simulink model "Sys1"  (R2017b)
settings: Solver=VariableStepAuto  StartTime=0.0  StopTime=10.0  RelTol=1e-3
values from neighbouring files (symbols this model uses):
  Gs_Ident = tf([-0.01542 5.826],[1 1.226])    [main.m]
libraries: simulink x1
settings Model: Creator=felip  LastModifiedBy=felip

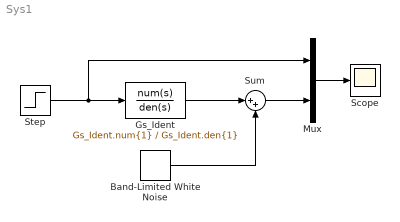
== system Sys1 ==
  Band-Limited White Noise : simulink/Sources/Band-Limited White Noise  Cov=1e-7  Ts=1e-3  seed=[23341]
  Gs_Ident : TransferFcn  Numerator=Gs_Ident.num{1}  Denominator=Gs_Ident.den{1}
  Mux : Mux  Inputs=2
  Scope : Scope
  Step : Step  SampleTime=0
  Sum : Sum  Inputs=|++
  wires:
  Step/1 -> Mux/1, Gs_Ident/1
  Gs_Ident/1 -> Sum/1
  Band-Limited White Noise/1 -> Sum/2
  Sum/1 -> Mux/2
  Mux/1 -> Scope/1
